simulink model "Power_consumption_simulation"  (R2019b)
settings: Solver=ode4  StartTime=0.0  StopTime=SIM_TIME  FixedStep=STEP_SIZE  RelTol=1e-3
values from neighbouring files (symbols this model uses):
  AD = 2.05    [Energy_budget_2020-05-07.m]
  CD = 0.2    [Energy_budget_2020-05-07.m]
  Crr = 0.006    [Energy_budget_2020-05-07.m]
  Fg = m_total*g    (= 7779.33)    [Energy_budget_2020-05-07.m]
  m_total = m_car + n_passenger*m_passenger    (= 793)    [Energy_budget_2020-05-07.m]
  r_wheel = 0.7/2    (= 0.35)    [Energy_budget_2020-05-07.m]
  rho = 1.184    [Energy_budget_2020-05-07.m]
undefined symbols (not defined in the file or in its folder): a, road_tilt, SIM_TIME, t1, TRAVLE_DISTANCE, TRAVLE_TIME
settings Model: Creator=chris_000  LastModifiedBy=chris_000

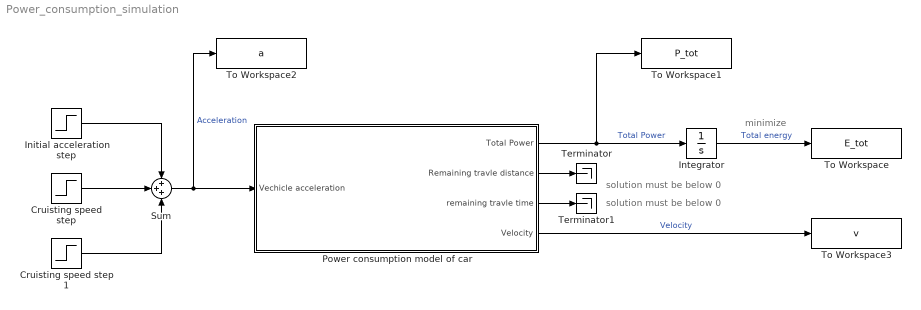
== system Power_consumption_simulation ==
  note: solution must be below 0
  note: solution must be below 0
  note: minimize
  "Cruisting speed step " : Step  Time=t1  After=-a  SampleTime=0
  Cruisting speed step 1 : Step  Time=SIM_TIME-t1  After=-a  SampleTime=0
  Initial acceleration step : Step  Time=0  After=a  SampleTime=0
  Integrator : Integrator
  Power consumption model of car : Subsystem
  Sum : Sum  Inputs=+++
  Terminator : Terminator
  Terminator1 : Terminator
  To Workspace : ToWorkspace  VariableName=E_tot  SaveFormat=Timeseries  SampleTime=-1
  To Workspace1 : ToWorkspace  VariableName=P_tot  SaveFormat=Timeseries  SampleTime=-1
  To Workspace2 : ToWorkspace  VariableName=a  SaveFormat=Timeseries  SampleTime=-1
  To Workspace3 : ToWorkspace  VariableName=v  SaveFormat=Timeseries  SampleTime=-1
  wires:
  Sum/1 -> To Workspace2/1, Power consumption model of car/1(Vechicle acceleration)  "Acceleration"
  Power consumption model of car/1(Total Power) -> To Workspace1/1, Integrator/1  "Total Power"
  Integrator/1 -> To Workspace/1  "Total energy"
  "Cruisting speed step "/1 -> Sum/2
  Initial acceleration step/1 -> Sum/1
  Cruisting speed step 1/1 -> Sum/3
  Power consumption model of car/2(Remaining travle distance) -> Terminator/1
  Power consumption model of car/3(remaining travle time) -> Terminator1/1
  Power consumption model of car/4("Velocity ") -> To Workspace3/1  "Velocity"

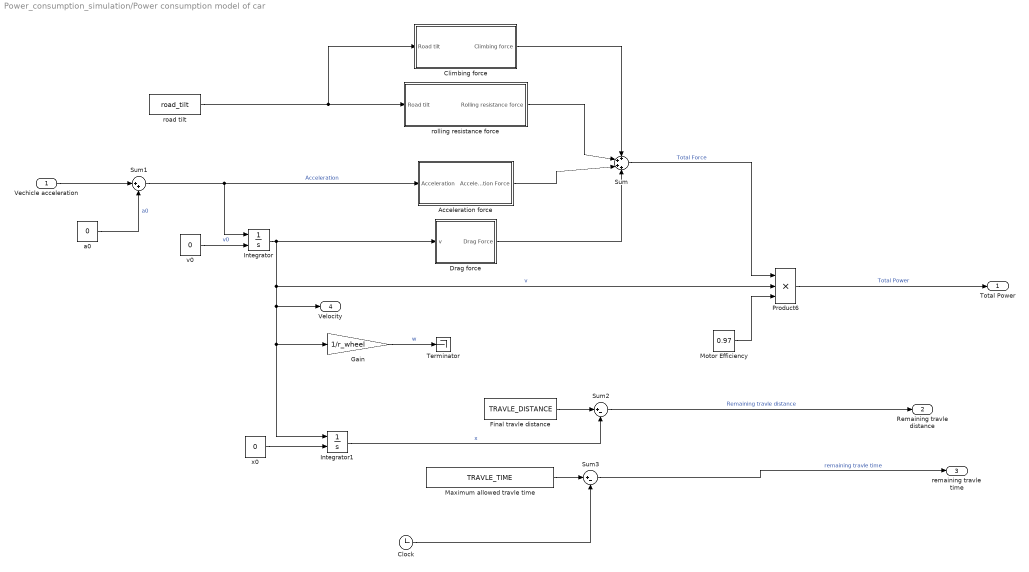
== system Power_consumption_simulation/Power consumption model of car ==
  Vechicle acceleration : Inport
  Acceleration force : Subsystem
  Climbing force : Subsystem
  Clock : Clock
      settings: Decimation=STEP_SIZE
  Drag force : Subsystem
  Final travle distance : Constant  Value=TRAVLE_DISTANCE
  Gain : Gain  Gain=1/r_wheel
  Integrator : Integrator  InitialConditionSource=external
  Integrator1 : Integrator  InitialConditionSource=external
  Maximum allowed travle time : Constant  Value=TRAVLE_TIME
  Motor Efficiency : Constant  Value=0.97
  Product6 : Product  Inputs=3
  Sum : Sum  Inputs=++++
  Sum1 : Sum  Inputs=|++
  Sum2 : Sum  Inputs=|+-
  Sum3 : Sum  Inputs=|+-
  Terminator : Terminator
  a0 : Constant  Value=0
  road tilt : Constant  Value=road_tilt
  rolling resistance force : Subsystem
  "v0 " : Constant  Value=0
  "x0 " : Constant  Value=0
  Total Power : Outport
  Remaining travle distance : Outport  Port=2
  remaining travle time : Outport  Port=3
  "Velocity " : Outport  Port=4
  wires:
  "x0 "/1 -> Integrator1/2
  Acceleration force/1(Acceleration Force) -> Sum/3
  Final travle distance/1 -> Sum2/1
  road tilt/1 -> Climbing force/1(Road tilt), rolling resistance force/1(Road tilt)
  Sum1/1 -> Integrator/1, Acceleration force/1(Acceleration)  "Acceleration"
  Product6/1 -> Total Power/1  "Total Power"
  Integrator/1 -> Drag force/1(v), "Velocity "/1, Gain/1, Integrator1/1, Product6/2  "v"
  Drag force/1(Drag Force) -> Sum/4
  Motor Efficiency/1 -> Product6/3
  Sum/1 -> Product6/1  "Total Force"
  Climbing force/1(Climbing force) -> Sum/1
  Integrator1/1 -> Sum2/2  "x"
  Gain/1 -> Terminator/1  "w"
  "v0 "/1 -> Integrator/2  "v0"
  a0/1 -> Sum1/2  "a0"
  Clock/1 -> Sum3/2
  rolling resistance force/1(Rolling resistance force) -> Sum/2
  Maximum allowed travle time/1 -> Sum3/1
  Vechicle acceleration/1 -> Sum1/1
  Sum2/1 -> Remaining travle distance/1  "Remaining travle distance"
  Sum3/1 -> remaining travle time/1  "remaining travle time"

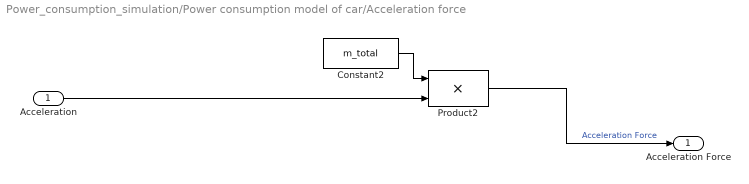
== system Power_consumption_simulation/Power consumption model of car/Acceleration force ==
  Acceleration : Inport
  Constant2 : Constant  Value=m_total
  Product2 : Product
  Acceleration Force : Outport
  wires:
  Constant2/1 -> Product2/1
  Product2/1 -> Acceleration Force/1  "Acceleration Force"
  Acceleration/1 -> Product2/2

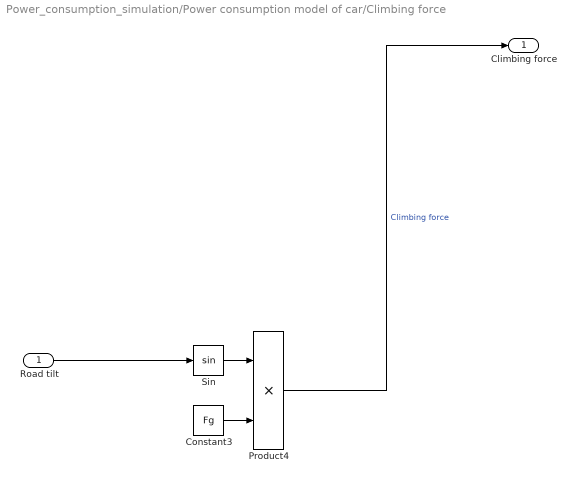
== system Power_consumption_simulation/Power consumption model of car/Climbing force ==
  Road tilt : Inport
  Constant3 : Constant  Value=Fg
  Product4 : Product
  Sin : Trigonometry
  Climbing force : Outport
  wires:
  Road tilt/1 -> Sin/1
  Constant3/1 -> Product4/2
  Sin/1 -> Product4/1
  Product4/1 -> Climbing force/1  "Climbing force"

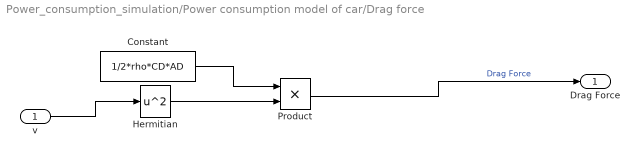
== system Power_consumption_simulation/Power consumption model of car/Drag force ==
  v : Inport
  Constant : Constant  Value=1/2*rho*CD*AD
  Hermitian : Math  Operator=square  SignedPower=off  SaturateOnIntegerOverflow=on
  Product : Product
  Drag Force : Outport
  wires:
  Product/1 -> Drag Force/1  "Drag Force"
  Hermitian/1 -> Product/2
  Constant/1 -> Product/1
  v/1 -> Hermitian/1

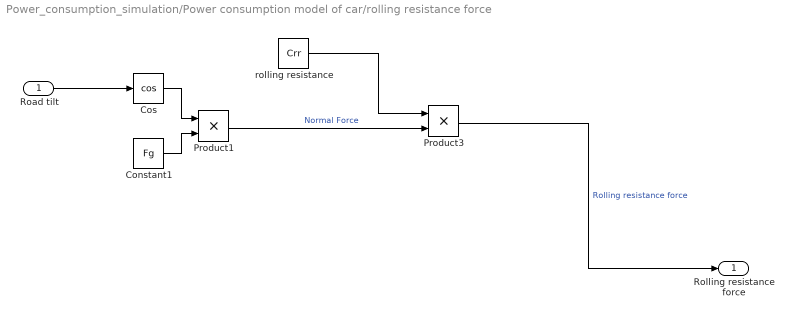
== system Power_consumption_simulation/Power consumption model of car/rolling resistance force ==
  Road tilt : Inport
  Constant1 : Constant  Value=Fg
  Cos : Trigonometry  Operator=cos
  Product1 : Product
  Product3 : Product
  "rolling resistance " : Constant  Value=Crr
  Rolling resistance force : Outport
  wires:
  Constant1/1 -> Product1/2
  Product3/1 -> Rolling resistance force/1  "Rolling resistance force"
  Cos/1 -> Product1/1
  Product1/1 -> Product3/2  "Normal Force"
  "rolling resistance "/1 -> Product3/1
  Road tilt/1 -> Cos/1
